simulink model "PID_ADRC_v2"  (R2022a)
settings: Solver=VariableStepAuto  StartTime=0.0  StopTime=15  RelTol=1e-3
InitFcn:
  | T_set=2;
  | b0=1/(13.1);
  | T_sam=0.003;
  | s_cl=-6/T_set;
  | s_eso=1.5*s_cl;
  | z_eso=exp(s_eso*T_sam);
  | Kd=-2*s_cl;
  | Kp=(s_cl)^2;
  | l1=-3*s_eso;
  | l2=3*(s_eso)^2;
  | l3=-(s_eso)^3;
  | 
  | 
  | %Thong so Notch filter
  | w0=4.337;
  | D=0.0001;
  | T_set1=3;
  | b01=1/(0.87);
  | T_sam1=0.003;
  | s_cl1=-6/T_set1;
  | s_eso1=20*s_cl1;
  | z_eso1=exp(s_eso1*T_sam1);
  | Kd1=-2*s_cl1;
  | Kp1=(s_cl1)^2;
  | l11=-3*s_eso1;
  | l21=3*(s_eso1)^2;
  | l31=-(s_eso1)^3;
libraries: slpidlib x2
settings Model: Creator=ducdu  LastModifiedBy=ducdu
settings DebuggingCC: UnderSpecifiedDimensionMsg=warning

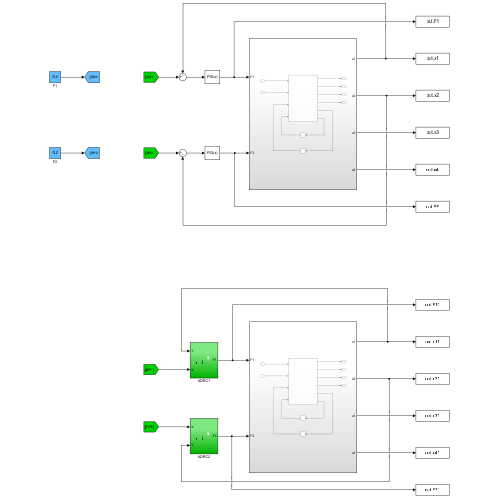
[thumbnail: Simulink's stored preview of the top-level diagram]
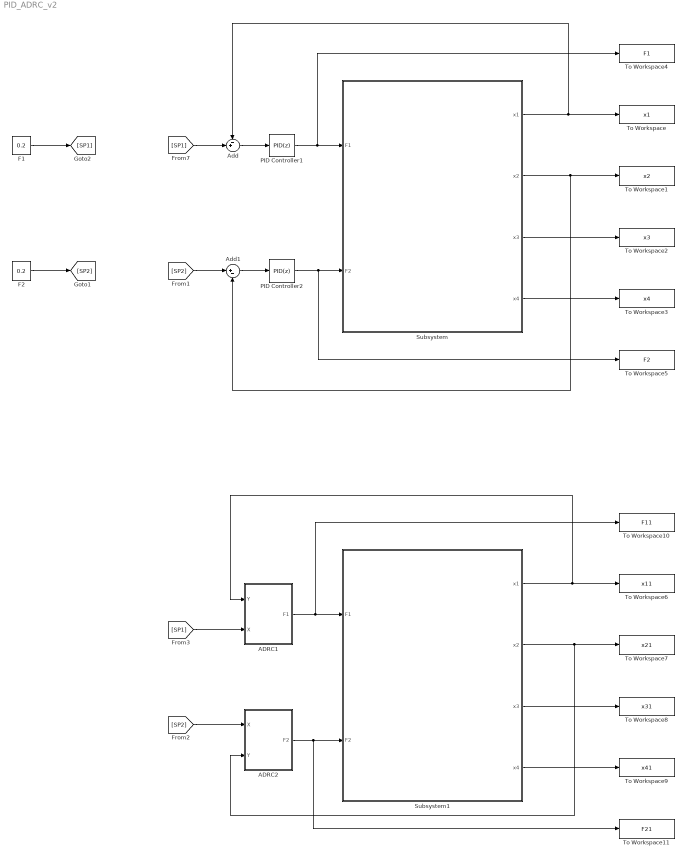
== system PID_ADRC_v2 ==
  ADRC1 : Subsystem
  ADRC2 : Subsystem
  Add : Sum  Inputs=-+|
  Add1 : Sum  Inputs=|+-
  F1 : Constant  Value=0.2
  F2 : Constant  Value=0.2
  PID Controller1 : slpidlib/PID Controller  Controller=PID  Form=Parallel  TimeDomain=Discrete-time  UseExternalTs=off  SampleTime=0.003  IntegratorMethod=Forward Euler  FilterMethod=Forward Euler  ControllerParametersSource=internal  P=0.18380080341484  I=0.00264427661684036  UseKiTs=off  D=14.3583596221209  N=105.481990683281  UseFilter=on  TunerSelectOption=Transfer Function Based (PID Tuner App)  InitialConditionSource=internal  InitialConditionForIntegrator=0  InitialConditionForFilter=0  DifferentiatorICPrevScaledInput=0  ExternalReset=none  TrackingMode=off  Kt=1  LimitOutput=off  SatLimitsSource=internal  UpperSaturationLimit=inf  LowerSaturationLimit=-inf  LinearizeAsGain=on  AntiWindupMode=none  Kb=1  POutMin=[]  POutMax=[]  IOutMin=[]  IOutMax=[]  DOutMin=[]  DOutMax=[]  NOutMin=[]  NOutMax=[]  SumOutMin=[]  SumOutMax=[]  SaturationOutMin=[]  SaturationOutMax=[]  PParamMin=[]  PParamMax=[]  IParamMin=[]  IParamMax=[]  DParamMin=[]  DParamMax=[]  NParamMin=[]  NParamMax=[]  KbParamMin=[]  KbParamMax=[]  KtParamMin=[]  KtParamMax=[]  KbOutMin=[]  KbOutMax=[]  KtOutMin=[]  KtOutMax=[]  IntegratorOutMin=[]  IntegratorOutMax=[]  FilterOutMin=[]  FilterOutMax=[]  SumI1OutMin=[]  SumI1OutMax=[]  SumI2OutMin=[]  SumI2OutMax=[]  SumI3OutMin=[]  SumI3OutMax=[]  SumI4OutMin=[]  SumI4OutMax=[]  SumDOutMin=[]  SumDOutMax=[]  DifferentiatorOutMin=[]  DifferentiatorOutMax=[]  FilterDiffOutCoefMin=[]  FilterDiffOutCoefMax=[]  ReciprocalOutMin=[]  ReciprocalOutMax=[]  SumDenOutMin=[]  SumDenOutMax=[]  SumNumOutMin=[]  SumNumOutMax=[]  DivideOutMin=[]  DivideOutMax=[]  UdiffTsProdOutMin=[]  UdiffTsProdOutMax=[]  NTsProdOutMin=[]  NTsProdOutMax=[]  UintegralTsProdOutMin=[]  UintegralTsProdOutMax=[]  UngainTsProdOutMin=[]  UngainTsProdOutMax=[]  IntegratorContinuousStateAttributes=''  IntegratorStateMustResolveToSignalObject=off  IntegratorRTWStateStorageClass=Auto  FilterContinuousStateAttributes=''  FilterStateMustResolveToSignalObject=off  FilterRTWStateStorageClass=Auto  ParallelPVariant=InternalParameters  IdealPVariant=Disabled  IVariant=InternalParameters  DVariant=InternalParameters  IntegratorVariant=Discrete  SatVariant=Disabled  AWVariant=Passthrough  PCopyVariant=Disabled  TRVariant=Disabled  FdbkBlocksVariant=Forward  IdealPFdbkVariant=Disabled  SatFdbkVariant=Disabled  DerivativeFilterVariant=ForwardEulerFilter  NVariant=InternalParameters  NCopyVariant=Disabled  FilterICVariant=InternalICsFilter  IntegratorICVariant=InternalICs  ExternalResetVariant=Disabled  TRSumVariant=Passthrough  SumFdbkVariant=Disabled  SumVariant=Sum_PID  TsampFilterVariant=InternalTs  TsampNgainVariant=Passthrough  TsampIntegralVariant=Passthrough  ExternalSaturationOutDataTypeStr=Inherit: Same as second input  aMode=0
  PID Controller2 : slpidlib/PID Controller  Controller=PID  Form=Parallel  TimeDomain=Discrete-time  UseExternalTs=off  SampleTime=0.003  IntegratorMethod=Forward Euler  FilterMethod=Forward Euler  ControllerParametersSource=internal  P=0.18380080341484  I=0.00264427661684036  UseKiTs=off  D=14.3583596221209  N=105.481990683281  UseFilter=on  TunerSelectOption=Transfer Function Based (PID Tuner App)  InitialConditionSource=internal  InitialConditionForIntegrator=0  InitialConditionForFilter=0  DifferentiatorICPrevScaledInput=0  ExternalReset=none  TrackingMode=off  Kt=1  LimitOutput=off  SatLimitsSource=internal  UpperSaturationLimit=inf  LowerSaturationLimit=-inf  LinearizeAsGain=on  AntiWindupMode=none  Kb=1  POutMin=[]  POutMax=[]  IOutMin=[]  IOutMax=[]  DOutMin=[]  DOutMax=[]  NOutMin=[]  NOutMax=[]  SumOutMin=[]  SumOutMax=[]  SaturationOutMin=[]  SaturationOutMax=[]  PParamMin=[]  PParamMax=[]  IParamMin=[]  IParamMax=[]  DParamMin=[]  DParamMax=[]  NParamMin=[]  NParamMax=[]  KbParamMin=[]  KbParamMax=[]  KtParamMin=[]  KtParamMax=[]  KbOutMin=[]  KbOutMax=[]  KtOutMin=[]  KtOutMax=[]  IntegratorOutMin=[]  IntegratorOutMax=[]  FilterOutMin=[]  FilterOutMax=[]  SumI1OutMin=[]  SumI1OutMax=[]  SumI2OutMin=[]  SumI2OutMax=[]  SumI3OutMin=[]  SumI3OutMax=[]  SumI4OutMin=[]  SumI4OutMax=[]  SumDOutMin=[]  SumDOutMax=[]  DifferentiatorOutMin=[]  DifferentiatorOutMax=[]  FilterDiffOutCoefMin=[]  FilterDiffOutCoefMax=[]  ReciprocalOutMin=[]  ReciprocalOutMax=[]  SumDenOutMin=[]  SumDenOutMax=[]  SumNumOutMin=[]  SumNumOutMax=[]  DivideOutMin=[]  DivideOutMax=[]  UdiffTsProdOutMin=[]  UdiffTsProdOutMax=[]  NTsProdOutMin=[]  NTsProdOutMax=[]  UintegralTsProdOutMin=[]  UintegralTsProdOutMax=[]  UngainTsProdOutMin=[]  UngainTsProdOutMax=[]  IntegratorContinuousStateAttributes=''  IntegratorStateMustResolveToSignalObject=off  IntegratorRTWStateStorageClass=Auto  FilterContinuousStateAttributes=''  FilterStateMustResolveToSignalObject=off  FilterRTWStateStorageClass=Auto  ParallelPVariant=InternalParameters  IdealPVariant=Disabled  IVariant=InternalParameters  DVariant=InternalParameters  IntegratorVariant=Discrete  SatVariant=Disabled  AWVariant=Passthrough  PCopyVariant=Disabled  TRVariant=Disabled  FdbkBlocksVariant=Forward  IdealPFdbkVariant=Disabled  SatFdbkVariant=Disabled  DerivativeFilterVariant=ForwardEulerFilter  NVariant=InternalParameters  NCopyVariant=Disabled  FilterICVariant=InternalICsFilter  IntegratorICVariant=InternalICs  ExternalResetVariant=Disabled  TRSumVariant=Passthrough  SumFdbkVariant=Disabled  SumVariant=Sum_PID  TsampFilterVariant=InternalTs  TsampNgainVariant=Passthrough  TsampIntegralVariant=Passthrough  ExternalSaturationOutDataTypeStr=Inherit: Same as second input  aMode=0
  Subsystem : Subsystem
  Subsystem1 : Subsystem
  To Workspace : ToWorkspace  VariableName=x1  SaveFormat=Timeseries  SampleTime=-1
  To Workspace1 : ToWorkspace  VariableName=x2  SaveFormat=Timeseries  SampleTime=-1
  To Workspace10 : ToWorkspace  VariableName=F11  SaveFormat=Timeseries  SampleTime=-1
  To Workspace11 : ToWorkspace  VariableName=F21  SaveFormat=Timeseries  SampleTime=-1
  To Workspace2 : ToWorkspace  VariableName=x3  SaveFormat=Timeseries  SampleTime=-1
  To Workspace3 : ToWorkspace  VariableName=x4  SaveFormat=Timeseries  SampleTime=-1
  To Workspace4 : ToWorkspace  VariableName=F1  SaveFormat=Timeseries  SampleTime=-1
  To Workspace5 : ToWorkspace  VariableName=F2  SaveFormat=Timeseries  SampleTime=-1
  To Workspace6 : ToWorkspace  VariableName=x11  SaveFormat=Timeseries  SampleTime=-1
  To Workspace7 : ToWorkspace  VariableName=x21  SaveFormat=Timeseries  SampleTime=-1
  To Workspace8 : ToWorkspace  VariableName=x31  SaveFormat=Timeseries  SampleTime=-1
  To Workspace9 : ToWorkspace  VariableName=x41  SaveFormat=Timeseries  SampleTime=-1
  wires:
  F1/1 -> [SP1]
  [SP1] -> Add/2
  PID Controller1/1 -> To Workspace4/1, Subsystem/1(F1)
  Add/1 -> PID Controller1/1
  F2/1 -> [SP2]
  Add1/1 -> PID Controller2/1
  PID Controller2/1 -> To Workspace5/1, Subsystem/2(F2)
  Subsystem/1(x1) -> To Workspace/1, Add/1
  Subsystem/2(x2) -> To Workspace1/1, Add1/2
  Subsystem/3(x3) -> To Workspace2/1
  Subsystem/4(x4) -> To Workspace3/1
  Subsystem1/4(x4) -> To Workspace9/1
  Subsystem1/2(x2) -> ADRC2/2(Y), To Workspace7/1
  Subsystem1/3(x3) -> To Workspace8/1
  Subsystem1/1(x1) -> ADRC1/1(Y), To Workspace6/1
  [SP1] -> ADRC1/2(X)
  ADRC1/1(F1) -> To Workspace10/1, Subsystem1/1(F1)
  [SP2] -> ADRC2/1(X)
  ADRC2/1(F2) -> To Workspace11/1, Subsystem1/2(F2)
  [SP2] -> Add1/1

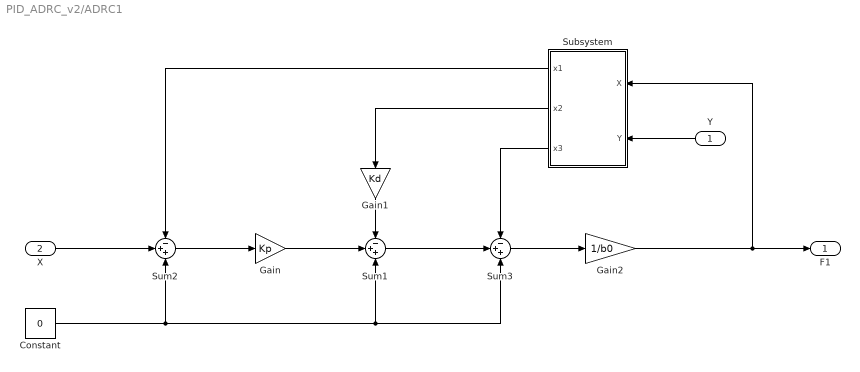
== system PID_ADRC_v2/ADRC1 ==
  Y : Inport
  X : Inport  Port=2
  Constant : Constant  Value=0
  Gain : Gain  Gain=Kp
  Gain1 : Gain  Gain=Kd
  Gain2 : Gain  Gain=1/b0
  Subsystem : Subsystem
  Sum1 : Sum  Inputs=-++
  Sum2 : Sum  Inputs=-++
  Sum3 : Sum  Inputs=-++
  F1 : Outport
  wires:
  Subsystem/1(x1) -> Sum2/1
  Sum3/1 -> Gain2/1
  Subsystem/3(x3) -> Sum3/1
  Gain2/1 -> F1/1, Subsystem/1(X)
  Subsystem/2(x2) -> Gain1/1
  Sum2/1 -> Gain/1
  Y/1 -> Subsystem/2(Y)
  X/1 -> Sum2/2
  Sum1/1 -> Sum3/2
  Gain1/1 -> Sum1/1
  Gain/1 -> Sum1/2
  Constant/1 -> Sum2/3, Sum1/3, Sum3/3

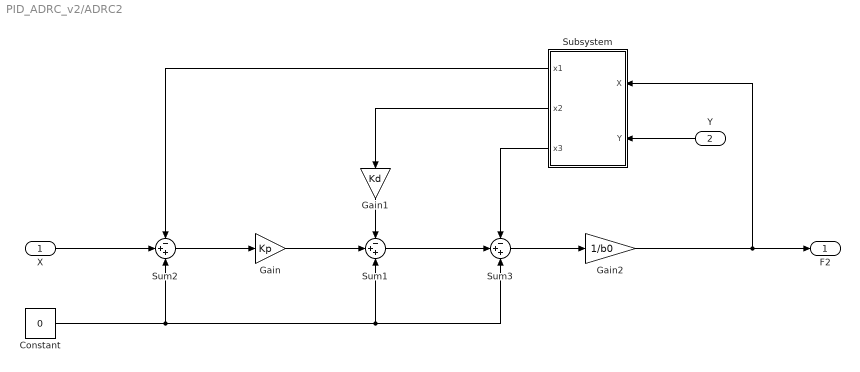
== system PID_ADRC_v2/ADRC2 ==
  X : Inport
  Y : Inport  Port=2
  Constant : Constant  Value=0
  Gain : Gain  Gain=Kp
  Gain1 : Gain  Gain=Kd
  Gain2 : Gain  Gain=1/b0
  Subsystem : Subsystem
  Sum1 : Sum  Inputs=-++
  Sum2 : Sum  Inputs=-++
  Sum3 : Sum  Inputs=-++
  F2 : Outport
  wires:
  Subsystem/1(x1) -> Sum2/1
  Sum3/1 -> Gain2/1
  Subsystem/3(x3) -> Sum3/1
  Gain2/1 -> F2/1, Subsystem/1(X)
  Subsystem/2(x2) -> Gain1/1
  Sum2/1 -> Gain/1
  Y/1 -> Subsystem/2(Y)
  X/1 -> Sum2/2
  Sum1/1 -> Sum3/2
  Gain1/1 -> Sum1/1
  Gain/1 -> Sum1/2
  Constant/1 -> Sum2/3, Sum1/3, Sum3/3

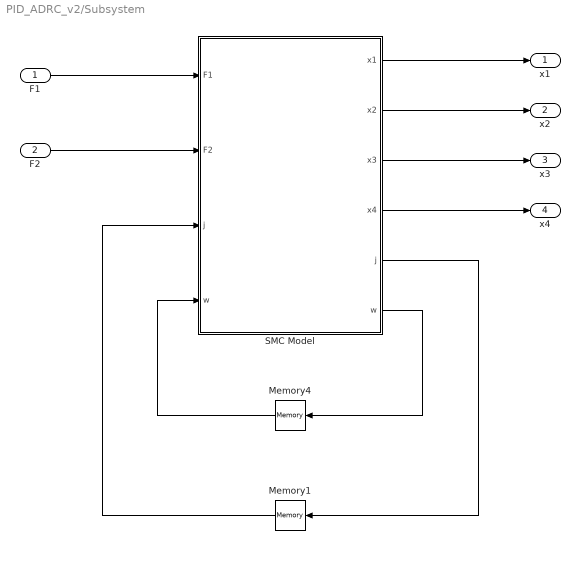
== system PID_ADRC_v2/Subsystem ==
  F1 : Inport
  F2 : Inport  Port=2
  Memory1 : Memory
  Memory4 : Memory  InitialCondition=zeros(15,20000)
  SMC Model : MATLAB Function  TreatAsAtomicUnit=on
  x1 : Outport
  x2 : Outport  Port=2
  x3 : Outport  Port=3
  x4 : Outport  Port=4
  wires:
  F1/1 -> SMC Model/1(F1)
  SMC Model/6(w) -> Memory4/1
  Memory1/1 -> SMC Model/3("j ")
  SMC Model/2(x2) -> x2/1
  SMC Model/5(j) -> Memory1/1
  SMC Model/1(x1) -> x1/1
  F2/1 -> SMC Model/2(F2)
  Memory4/1 -> SMC Model/4("w ")
  SMC Model/3(x3) -> x3/1
  SMC Model/4(x4) -> x4/1

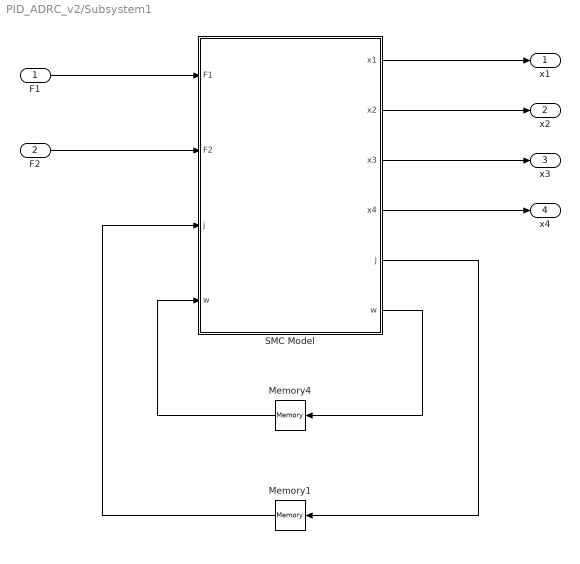
== system PID_ADRC_v2/Subsystem1 ==
  F1 : Inport
  F2 : Inport  Port=2
  Memory1 : Memory
  Memory4 : Memory  InitialCondition=zeros(20,20000)
  SMC Model : MATLAB Function  TreatAsAtomicUnit=on
  x1 : Outport
  x2 : Outport  Port=2
  x3 : Outport  Port=3
  x4 : Outport  Port=4
  wires:
  F1/1 -> SMC Model/1(F1)
  SMC Model/6(w) -> Memory4/1
  Memory1/1 -> SMC Model/3("j ")
  SMC Model/2(x2) -> x2/1
  SMC Model/5(j) -> Memory1/1
  SMC Model/1(x1) -> x1/1
  F2/1 -> SMC Model/2(F2)
  Memory4/1 -> SMC Model/4("w ")
  SMC Model/3(x3) -> x3/1
  SMC Model/4(x4) -> x4/1

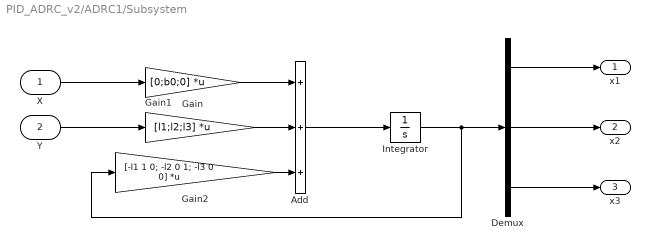
== system PID_ADRC_v2/ADRC1/Subsystem ==
  X : Inport
  Y : Inport  Port=2
  Add : Sum  Inputs=+++
  Demux : Demux  Outputs=3
  Gain : Gain  Gain=[0;b0;0]  Multiplication=Matrix(K*u)
  Gain1 : Gain  Gain=[l1;l2;l3]  Multiplication=Matrix(K*u)
  Gain2 : Gain  Gain=[-l1 1 0; -l2 0 1; -l3 0 0]  Multiplication=Matrix(K*u)
  Integrator : Integrator
  x1 : Outport
  x2 : Outport  Port=2
  x3 : Outport  Port=3
  wires:
  Gain1/1 -> Add/2
  Demux/3 -> x3/1
  Demux/1 -> x1/1
  Gain2/1 -> Add/3
  Demux/2 -> x2/1
  Gain/1 -> Add/1
  Add/1 -> Integrator/1
  Integrator/1 -> Gain2/1, Demux/1
  Y/1 -> Gain1/1
  X/1 -> Gain/1

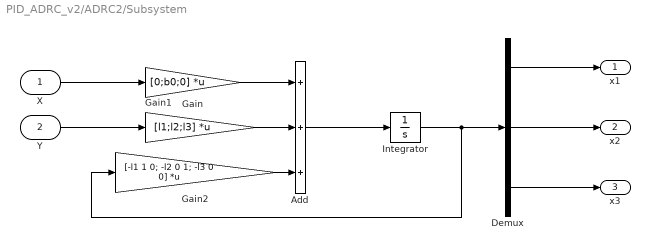
== system PID_ADRC_v2/ADRC2/Subsystem ==
  X : Inport
  Y : Inport  Port=2
  Add : Sum  Inputs=+++
  Demux : Demux  Outputs=3
  Gain : Gain  Gain=[0;b0;0]  Multiplication=Matrix(K*u)
  Gain1 : Gain  Gain=[l1;l2;l3]  Multiplication=Matrix(K*u)
  Gain2 : Gain  Gain=[-l1 1 0; -l2 0 1; -l3 0 0]  Multiplication=Matrix(K*u)
  Integrator : Integrator
  x1 : Outport
  x2 : Outport  Port=2
  x3 : Outport  Port=3
  wires:
  Gain1/1 -> Add/2
  Demux/3 -> x3/1
  Demux/1 -> x1/1
  Gain2/1 -> Add/3
  Demux/2 -> x2/1
  Gain/1 -> Add/1
  Add/1 -> Integrator/1
  Integrator/1 -> Gain2/1, Demux/1
  Y/1 -> Gain1/1
  X/1 -> Gain/1

== matlab function PID_ADRC_v2/Subsystem1/SMC Model ==
  data: F1 input; F2 input; j input; w input; x1 output; x2 output; x3 output; x4 output; j output; w output
% 
function [x1,x2,x3,x4,j,w] = systemModeling(F1,F2,j,w)
    % Thiết lập các thông số cho dầm
    L = 0.63; EI = 0.754; rho_A = .297;
    % Các vật nặng 
    mw = 13.1; mk = 0.04; mh = 0.86; g = 9.81;
    
    % Thiết lập bước sai phân không gian và thời gian
    n = 9; r = 10000;
    tmax = 15;
    delta_Y = L/(n - 1); % Bước không gian
    delta_t = tmax/r; % Bước thời gian
    
    x3 = zeros(1,r);
    x2 = 2; 
    dx2dt_2 = zeros(1,r);
    dx2dt_2(1:3) = delta_Y;
    j = j + 1;
    
    %--------------------------------------------------------------------------
    wyyy0 = (w(3,j + 1) - 2*w(2,j + 1) + w(1,j + 1))/(2*delta_Y^3);
    S2 = (F1 - EI*wyyy0)/mw;
    w(1,j + 2) = 2*w(1,j + 1) - w(1,j) + delta_t^2*S2; % 5b
    w(2,j + 2) = w(1, j + 2);
    for i = 3:(n - 2)
        % Đạo hàm theo Y
        wyyyy = (w(i + 2,j + 1) - 4*w(i + 1,j + 1) + 6*w(i,j + 1) - 4*w(i - 1,j + 1) + w(i - 2,j + 1));
        S1 = (-EI/(rho_A*delta_Y^4))*wyyyy; 
        S4 = (-EI/(mh*delta_Y^3))*wyyyy;
    
        % Chuyển động của xe nâng
        dx3dt_2 = (x3(j + 2) - 2*x3(j + 1) + x3(j))/(2*delta_t^2);
        wyx2 = (w(x2 + 1,j) - w(x2 - 1,j))/(2*delta_Y^2);
        dx2dt_2(j + 2) = 2*dx2dt_2(j + 1) - dx2dt_2(j) + (F2 - mh*g - mh*dx3dt_2*wyx2)/mh*delta_t^2; % 5c
    
        % Cập nhật vị trí x2
        if dx2dt_2(j + 2) < delta_Y
            x2 = 2;
            dx2dt_2(j + 2) = delta_Y;
        elseif dx2dt_2(j + 2) > L - delta_Y
            x2 = n - 1;
            dx2dt_2(j + 2) = L - delta_Y;
        else
            x2 = ceil(dx2dt_2(j + 2)/delta_Y);
        end
    
        % Độ lắc của thanh
        if dx2dt_2(j + 2) ~= x2
            w(i,j + 2) = 2*w(i,j + 1) - w(i,j) + delta_t^2*S1; % 5a
            x3(j + 2) = w(i,j + 2) - w(1,j + 2);
        else
            w(i,j + 2) = 2*w(i,j + 1) - w(i,j) + delta_t^2*S4; % 5d
            x3(j + 2) = w(i,j + 2) - w(1,j + 2);
        end
    end
    wyyyl = (-2*w(n,j + 1) + 3*w(n - 1,j + 1) - w(n - 2,j + 1))/(2*delta_Y^3);
    S3 = (EI/mk)*wyyyl;
    w(n,j + 2) = 2*w(n,j + 1) - w(n,j) + delta_t^2*S3; % 5e
    w(n - 1,j + 2) = (w(n,j + 2) + w(n - 2,j + 2))/2;
    
    % Đầu ra
    x1 = w(1,j); % Vị trí xe con
    x2 = dx2dt_2(j); % Vị trí xe nâng
    x3 = x3(j); % Độ lắc xe nâng
    x4 = w(n,j) - w(1,j); % Độ lắc đỉnh thanh

end

== matlab function PID_ADRC_v2/Subsystem/SMC Model ==
  data: F1 input; F2 input; j input; w input; x1 output; x2 output; x3 output; x4 output; j output; w output
function [x1,x2,x3,x4,j,w] = systemModeling(F1,F2,j,w)
    % Thiết lập các thông số cho dầm
    L = 0.63; EI = 0.754; rho_A = .297;
    % Các vật nặng 
    mw = 13.1; mk = 0.04; mh = 0.86; g = 9.81;
    
    % Thiết lập bước sai phân không gian và thời gian
    n = 9; r = 10000;
    tmax = 15;
    delta_Y = L/(n - 1); % Bước không gian
    delta_t = tmax/r; % Bước thời gian
    
    x3 = zeros(1,r);
    x2 = 2; 
    dx2dt_2 = zeros(1,r);
    dx2dt_2(1:3) = delta_Y;
    j = j + 1;
    
    %--------------------------------------------------------------------------
    wyyy0 = (w(3,j + 1) - 2*w(2,j + 1) + w(1,j + 1))/(2*delta_Y^3);
    S2 = (F1 - EI*wyyy0)/mw;
    w(1,j + 2) = 2*w(1,j + 1) - w(1,j) + delta_t^2*S2; % 5b
    w(2,j + 2) = w(1, j + 2);
    for i = 3:(n - 2)
        % Đạo hàm theo Y
        wyyyy = (w(i + 2,j + 1) - 4*w(i + 1,j + 1) + 6*w(i,j + 1) - 4*w(i - 1,j + 1) + w(i - 2,j + 1));
        S1 = (-EI/(rho_A*delta_Y^4))*wyyyy; 
        S4 = (-EI/(mh*delta_Y^3))*wyyyy;
    
        % Chuyển động của xe nâng
        dx3dt_2 = (x3(j + 2) - 2*x3(j + 1) + x3(j))/(2*delta_t^2);
        wyx2 = (w(x2 + 1,j) - w(x2 - 1,j))/(2*delta_Y^2);
        dx2dt_2(j + 2) = 2*dx2dt_2(j + 1) - dx2dt_2(j) + (F2 - mh*g - mh*dx3dt_2*wyx2)/mh*delta_t^2; % 5c
    
        % Cập nhật vị trí x2
        if dx2dt_2(j + 2) < delta_Y
            x2 = 2;
            dx2dt_2(j + 2) = delta_Y;
        elseif dx2dt_2(j + 2) > L - delta_Y
            x2 = n - 1;
            dx2dt_2(j + 2) = L - delta_Y;
        else
            x2 = ceil(dx2dt_2(j + 2)/delta_Y);
        end
    
        % Độ lắc của thanh
        if dx2dt_2(j + 2) ~= x2
            w(i,j + 2) = 2*w(i,j + 1) - w(i,j) + delta_t^2*S1; % 5a
            x3(j + 2) = w(i,j + 2) - w(1,j + 2);
        else
            w(i,j + 2) = 2*w(i,j + 1) - w(i,j) + delta_t^2*S4; % 5d
            x3(j + 2) = w(i,j + 2) - w(1,j + 2);
        end
    end
    wyyyl = (-2*w(n,j + 1) + 3*w(n - 1,j + 1) - w(n - 2,j + 1))/(2*delta_Y^3);
    S3 = (EI/mk)*wyyyl;
    w(n,j + 2) = 2*w(n,j + 1) - w(n,j) + delta_t^2*S3; % 5e
    w(n - 1,j + 2) = (w(n,j + 2) + w(n - 2,j + 2))/2;
    
    % Đầu ra
    x1 = w(1,j); % Vị trí xe con
    x2 = dx2dt_2(j); % Vị trí xe nâng
    x3 = x3(j); % Độ lắc xe nâng
    x4 = w(n,j) - w(1,j); % Độ lắc đỉnh thanh

end
